simulink model "Aufgabe1"  (R2022b)
settings: Solver=VariableStepAuto  StartTime=0.0  StopTime=10  RelTol=1e-3
settings Model: Creator=psumMacWindows  LastModifiedBy=psumMacWindows

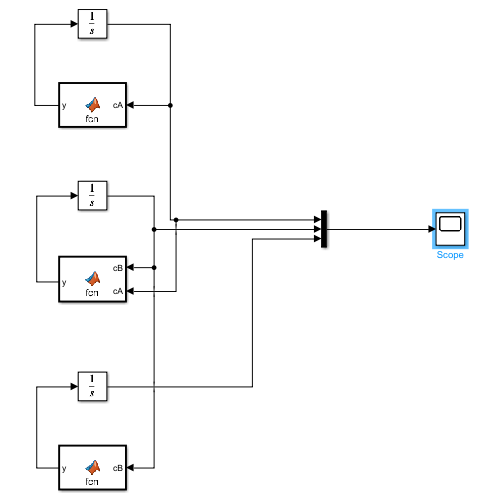
[thumbnail: Simulink's stored preview of the top-level diagram]
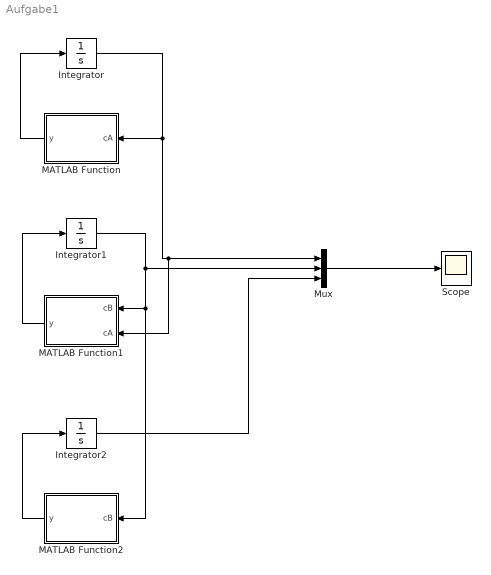
== system Aufgabe1 ==
  Integrator : Integrator  InitialCondition=1
  Integrator1 : Integrator
  Integrator2 : Integrator
  MATLAB Function : MATLAB Function  TreatAsAtomicUnit=on
  MATLAB Function1 : MATLAB Function  TreatAsAtomicUnit=on
  MATLAB Function2 : MATLAB Function  TreatAsAtomicUnit=on
  Mux : Mux  Inputs=3
  Scope : Scope
  wires:
  Integrator/1 -> MATLAB Function1/2(cA), Mux/1, MATLAB Function/1(cA)
  MATLAB Function/1(y) -> Integrator/1
  MATLAB Function1/1(y) -> Integrator1/1
  Integrator1/1 -> MATLAB Function2/1(cB), MATLAB Function1/1(cB), Mux/2
  MATLAB Function2/1(y) -> Integrator2/1
  Integrator2/1 -> Mux/3
  Mux/1 -> Scope/1

== matlab function Aufgabe1/MATLAB Function ==
  data: cA input; y output
function y = fcn(cA)

y = (-1) *cA;

== matlab function Aufgabe1/MATLAB Function2 ==
  data: cB input; y output
function y = fcn(cB)

y = 2*cB;

== matlab function Aufgabe1/MATLAB Function1 ==
  data: cB input; cA input; y output
function y = fcn(cB, cA)

y = cA-2*1*cB;
